simulink model "NDI_TSS_dynamics"  (R2024b)
settings: Solver=FixedStepAuto  StartTime=0.0  StopTime=1500  FixedStep=0.1  RelTol=1e-6  AbsTol=1e-6
values from neighbouring files (symbols this model uses):
  com_0 = [0,0,0]    [Specefications.m]
  com_1 = [60,60,60]*deg    [Specefications.m]
  com_2 = [-60,-60,-60]*deg    [Specefications.m]
  com_3 = [0,0,0]*deg    [Specefications.m]
  deg = pi/180    (= 0.0174532925199)    [Specefications.m]
  init_q = eul2quat(initial_euler_angles,"ZYX")    [Specefications.m]
  J = diag([J11,J22,J33])    [Specefications.m]
  K_o = lqr(A,B,Q,R)    [Linear_controller_design.m]
  n = (mu_Earth/r^3).^0.5    [Specefications.m]
  t_d = [1e-4,1e-4,1e-4]    [Specefications.m]
  w = [0,0,0].*deg    [Specefications.m]
libraries: matrix_library x3, aerolibutil x3, sharedtransform x1, sharedutil x1
settings Model: Creator=diogo  LastModifiedBy=diogo

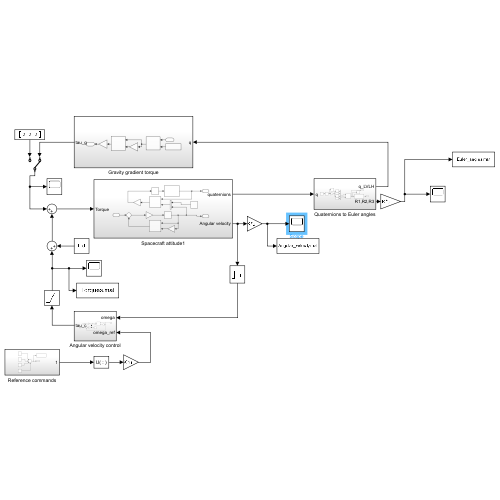
[thumbnail: Simulink's stored preview of the top-level diagram]
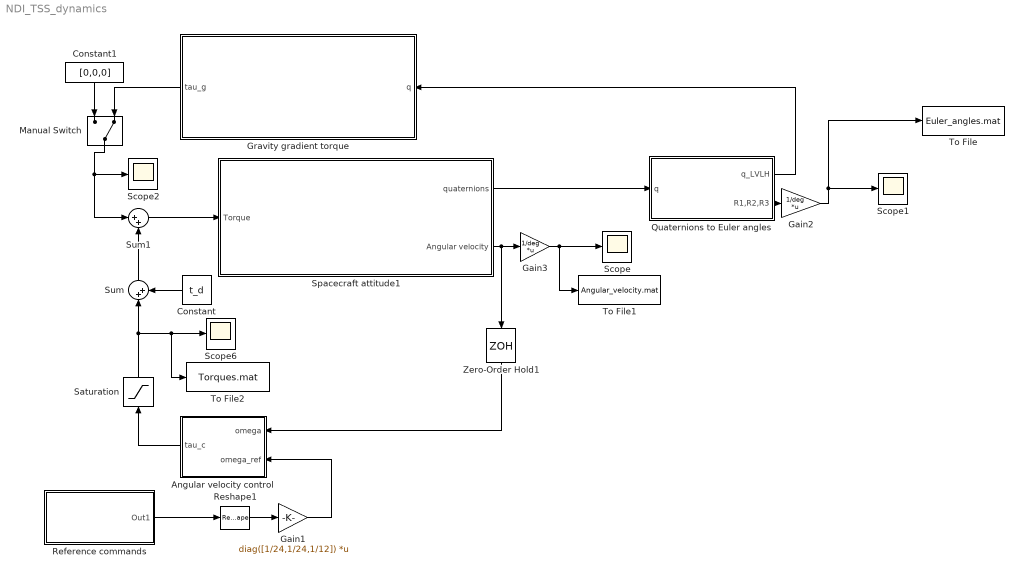
== system NDI_TSS_dynamics ==
  Angular velocity control : Subsystem
      settings: PortSchema="{\"entries\":[{\"content\":{\"sides\":[{\"content\":{\"connectorIds\":[\"Out1\"]},\"type\":\"ConnectorPlacement.EquallySpacedRectSide\",\"uuid\":\"1a2144e1-4a42-45d8-bf34-f3ce2743180d\"},{\"content\":{\"connectorIds\":[\"In1\",\"In2\"],\"side\":\"RIGHT\"},\"type\":\"ConnectorPlacement.EquallySpacedRectSide\",\"uuid\":\"d3edec84-6c6c-4d61-a4e7-efc1d8cfdc8e\"},{\"content\":{\"side\":\"TOP\"},\"type\":\"ConnectorPlacement.EquallySpacedRectSide\",\"uuid\":\"4603dd34-691c-41cc-8d1f-b520c222b747\"}]},\"type\":\"ConnectorPlacement.EquallySpacedConnector\",\"uuid\":\"cb96d0f2-f61f-49d9-873a-c73fce2fea98\"}],\"packageUris\":[\"http://schema.mathworks.com/mf0/Connector/R2020b\"],\"version\":\"1.0\"}"
  Constant : Constant  Value=t_d
  Constant1 : Constant  Value=[0,0,0]
  Gain1 : Gain  Gain=diag([1/24,1/24,1/12])  Multiplication=Matrix(K*u)
  Gain2 : Gain  Gain=1/deg  Multiplication=Matrix(K*u)
  Gain3 : Gain  Gain=1/deg  Multiplication=Matrix(K*u)
  Gravity gradient torque : Subsystem
  Manual Switch : ManualSwitch  CurrentSetting=0
  Quaternions to Euler angles : Subsystem
  Reference commands : Subsystem
  Reshape1 : Reshape
  Saturation : Saturate  UpperLimit=1.5  LowerLimit=-1.5
  Scope{,1..2,6} (4 alike) : Scope
  Spacecraft attitude1 : Subsystem
  Sum : Sum  Inputs=|++
  Sum1 : Sum  Inputs=|++
  To File : ToFile  Filename=Euler_angles.mat  MatrixName=values  SaveFormat=Timeseries
  To File1 : ToFile  Filename=Angular_velocity.mat  MatrixName=values  SaveFormat=Timeseries
  To File2 : ToFile  Filename=Torques.mat  MatrixName=values  SaveFormat=Timeseries
  Zero-Order Hold1 : ZeroOrderHold  SampleTime=0.1
  wires:
  Gain3/1 -> To File1/1, Scope/1
  Spacecraft attitude1/2(Angular velocity) -> Zero-Order Hold1/1, Gain3/1
  Constant/1 -> Sum/2
  Sum/1 -> Sum1/2
  Sum1/1 -> Spacecraft attitude1/1(Torque)
  Gain2/1 -> To File/1, Scope1/1
  Constant1/1 -> Manual Switch/1
  Gravity gradient torque/1(tau_g) -> Manual Switch/2
  Manual Switch/1 -> Sum1/1, Scope2/1
  Reference commands/1(Out1) -> Reshape1/1
  Saturation/1 -> Sum/1, To File2/1, Scope6/1
  Zero-Order Hold1/1 -> Angular velocity control/1(omega)
  Angular velocity control/1(tau_c) -> Saturation/1
  Reshape1/1 -> Gain1/1
  Gain1/1 -> Angular velocity control/2(omega_ref)
  Quaternions to Euler angles/2(R1,R2,R3) -> Gain2/1
  Spacecraft attitude1/1(quaternions) -> Quaternions to Euler angles/1(q)
  Quaternions to Euler angles/1(q_LVLH) -> Gravity gradient torque/1(q)

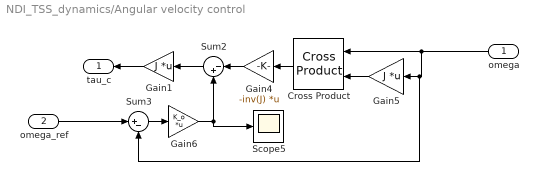
== system NDI_TSS_dynamics/Angular velocity control ==
  omega : Inport
  omega_ref : Inport  Port=2
  Cross Product : matrix_library/Cross Product
  Gain1 : Gain  Gain=J  Multiplication=Matrix(K*u)
  Gain4 : Gain  Gain=-inv(J)  Multiplication=Matrix(K*u)
  Gain5 : Gain  Gain=J  Multiplication=Matrix(K*u)
  Gain6 : Gain  Gain=K_o  Multiplication=Matrix(K*u)
  Scope5 : Scope
  Sum2 : Sum  Inputs=|-+
  Sum3 : Sum  Inputs=|+-
  tau_c : Outport
  wires:
  omega/1 -> Cross Product/1, Sum3/2, Gain5/1
  Sum2/1 -> Gain1/1
  Gain4/1 -> Sum2/1
  Cross Product/1 -> Gain4/1
  Gain6/1 -> Sum2/2, Scope5/1
  Gain1/1 -> tau_c/1
  Sum3/1 -> Gain6/1
  Gain5/1 -> Cross Product/2
  omega_ref/1 -> Sum3/1

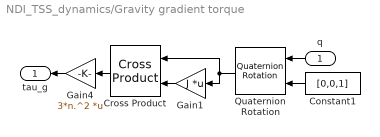
== system NDI_TSS_dynamics/Gravity gradient torque ==
  q : Inport
  Constant1 : Constant  Value=[0,0,1]
  Cross Product : matrix_library/Cross Product
  Gain1 : Gain  Gain=J  Multiplication=Matrix(K*u)
  Gain4 : Gain  Gain=3*n.^2  Multiplication=Matrix(K*u)
  Quaternion Rotation : aerolibutil/Quaternion Rotation
  tau_g : Outport
  wires:
  Constant1/1 -> Quaternion Rotation/2
  Gain1/1 -> Cross Product/2
  Quaternion Rotation/1 -> Gain1/1, Cross Product/1
  Gain4/1 -> tau_g/1
  Cross Product/1 -> Gain4/1
  q/1 -> Quaternion Rotation/1

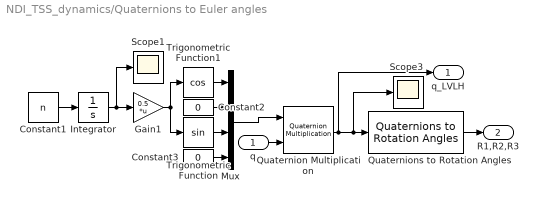
== system NDI_TSS_dynamics/Quaternions to Euler angles ==
  q : Inport
  Constant1 : Constant  Value=n
  Constant2 : Constant  Value=0
  Constant3 : Constant  Value=0
  Gain1 : Gain  Gain=0.5  Multiplication=Matrix(K*u)
  Integrator : Integrator
  Mux : Mux
  Quaternion Multiplication : aerolibutil/Quaternion Multiplication
  Quaternions to Rotation Angles : sharedtransform/Quaternions to Rotation Angles  rotationOrder=ZYX  aMode=aMode
  Scope1 : Scope
  Scope3 : Scope
  Trigonometric Function : Trigonometry
  Trigonometric Function1 : Trigonometry  Operator=cos
  q_LVLH : Outport
  R1,R2,R3 : Outport  Port=2
  wires:
  Gain1/1 -> Trigonometric Function1/1, Trigonometric Function/1
  Constant3/1 -> Mux/4
  Constant1/1 -> Integrator/1
  Quaternion Multiplication/1 -> q_LVLH/1, Scope3/1, Quaternions to Rotation Angles/1
  Integrator/1 -> Scope1/1, Gain1/1
  Constant2/1 -> Mux/2
  Trigonometric Function1/1 -> Mux/1
  Quaternions to Rotation Angles/1 -> R1,R2,R3/1
  Trigonometric Function/1 -> Mux/3
  Mux/1 -> Quaternion Multiplication/1
  q/1 -> Quaternion Multiplication/2

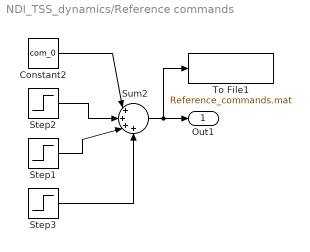
== system NDI_TSS_dynamics/Reference commands ==
  Constant2 : Constant  Value=com_0
  Step1 : Step  Time=500.1  After=com_2 - com_1  SampleTime=0  VectorParams1D=off
  Step2 : Step  Time=100  After=com_1 - com_0  SampleTime=0  VectorParams1D=off
  Step3 : Step  Time=900.1  After=com_3 - com_2  SampleTime=0  VectorParams1D=off
  Sum2 : Sum  Inputs=|++++
  To File1 : ToFile  Filename=Reference_commands.mat  MatrixName=values  SaveFormat=Timeseries
  Out1 : Outport
  wires:
  Step3/1 -> Sum2/4
  Step1/1 -> Sum2/3
  Step2/1 -> Sum2/2
  Constant2/1 -> Sum2/1
  Sum2/1 -> To File1/1, Out1/1

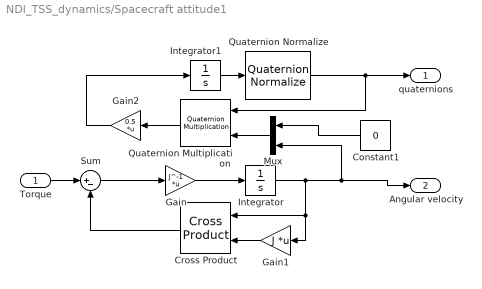
== system NDI_TSS_dynamics/Spacecraft attitude1 ==
  Torque : Inport
  Constant1 : Constant  Value=0
  Cross Product : matrix_library/Cross Product
  Gain : Gain  Gain=J^-1  Multiplication=Matrix(K*u)
  Gain1 : Gain  Gain=J  Multiplication=Matrix(K*u)
  Gain2 : Gain  Gain=0.5  Multiplication=Matrix(K*u)
  Integrator : Integrator  InitialCondition=w
  Integrator1 : Integrator  InitialCondition=init_q
  Mux : Mux  Inputs=2
  Quaternion Multiplication : aerolibutil/Quaternion Multiplication
  Quaternion Normalize : sharedutil/Quaternion Normalize  aMode=aMode
  Sum : Sum  Inputs=|+-
  quaternions : Outport
  Angular velocity : Outport  Port=2
  wires:
  Gain1/1 -> Cross Product/2
  Integrator/1 -> Cross Product/1, Gain1/1, Angular velocity/1, Mux/2
  Sum/1 -> Gain/1
  Cross Product/1 -> Sum/2
  Integrator1/1 -> Quaternion Normalize/1
  Gain/1 -> Integrator/1
  Mux/1 -> Quaternion Multiplication/2
  Quaternion Normalize/1 -> quaternions/1, Quaternion Multiplication/1
  Gain2/1 -> Integrator1/1
  Quaternion Multiplication/1 -> Gain2/1
  Constant1/1 -> Mux/1
  Torque/1 -> Sum/1
